simulink model "Virtual_Exhaust_Aftertreatment_System_Model"  (R2016b)
settings: Solver=FixedStepDiscrete  StartTime=0.0  StopTime=inf  FixedStep=VirtExhATSysMdl.tiSimnTiStep_C  RelTol=1e-3  EnableMultiTasking=on
undefined symbols (not defined in the file or in its folder): VirtExhATSysMdl
libraries: simulink x1
settings Model: Creator=m01wolf  LastModifiedBy=m01wolf
settings DataIOCC: SaveFormat=StructureWithTime  SaveOutput=off  DSMLogging=off  VisualizeSimOutput=off  SaveTime=off  SignalLoggingName=Results
settings OptimizationCC: BlockReduction=off  ConditionallyExecuteInputs=off  LifeSpan=inf
settings DebuggingCC: AllowSymbolicDim=off  SFUnexpectedBacktrackingDiag=warning  SFNoUnconditionalDefaultTransitionDiag=warning  SFExecutionAtInitializationDiag=none
settings ModelReferenceCC: ModelReferenceNumInstancesAllowed=Single  PropagateSignalLabelsOutOfModel=off
settings GRTTargetCC: TargetLangStandard=C89/C90 (ANSI)
settings ConfigComp: CovMetricSettings=dw  CovHtmlReporting=on  CovSaveCumulativeToWorkspaceVar=on  CovSaveSingleToWorkspaceVar=on  CovExternalEMLEnable=off

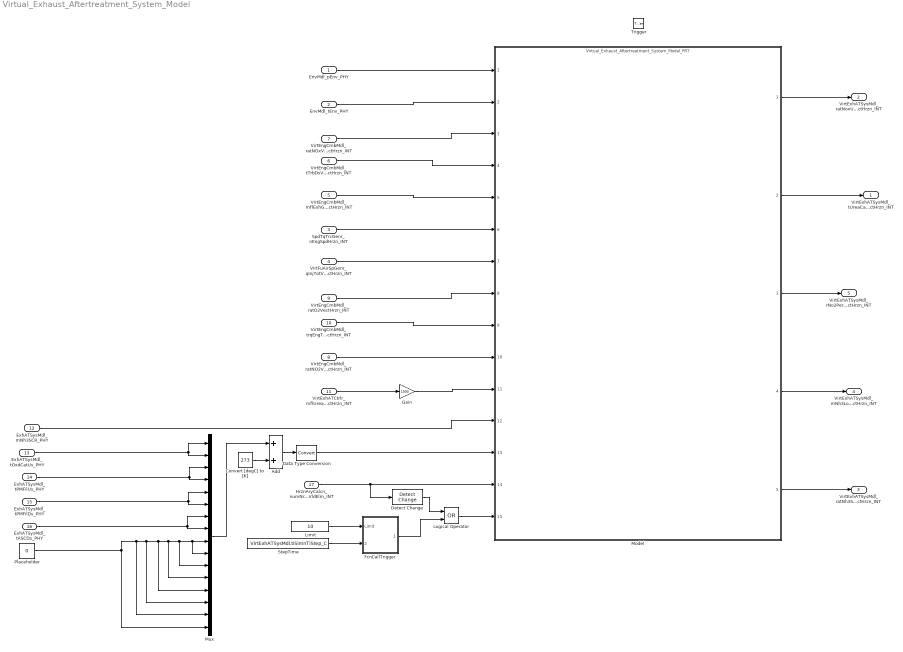
== system Virtual_Exhaust_Aftertreatment_System_Model ==
  EnvMdl_pEnv_PHY : Inport
  EnvMdl_tEnv_PHY : Inport  Port=2
  SpdTqTrcGenr_nEngSpdHrzn_INT : Inport  Port=3  PortDimensions=VirtExhATSysMdl_numHrznSize_CA
  VirtFuAirSpGenr_qInjTotVectHrzn_INT : Inport  Port=4  PortDimensions=VirtExhATSysMdl_numHrznSize_CA
  VirtEngCmbMdl_mflExhGasVectHrzn_INT : Inport  Port=5  PortDimensions=VirtExhATSysMdl_numHrznSize_CA
  VirtEngCmbMdl_tTrbDsVectHrzn_INT : Inport  Port=6  PortDimensions=VirtExhATSysMdl_numHrznSize_CA
  VirtEngCmbMdl_ratNOxVectHrzn_INT : Inport  Port=7  PortDimensions=VirtExhATSysMdl_numHrznSize_CA
  VirtEngCmbMdl_ratNO2VectHrzn_INT : Inport  Port=8  PortDimensions=VirtExhATSysMdl_numHrznSize_CA
  VirtEngCmbMdl_ratO2VectHrzn_INT : Inport  Port=9  PortDimensions=VirtExhATSysMdl_numHrznSize_CA
  VirtEngCmbMdl_trqEngTqOutVectHrzn_INT : Inport  Port=10  PortDimensions=VirtExhATSysMdl_numHrznSize_CA
  VirtExhATCtrlr_mflUreaDesVectHrzn_INT : Inport  Port=11  PortDimensions=VirtExhATSysMdl_numHrznSize_CA
  ExhATSysMdl_mNh3SCR_PHY : Inport  Port=12
  ExhATSysMdl_tOxdCatUs_PHY : Inport  Port=13
  ExhATSysMdl_tPMFilUs_PHY : Inport  Port=14
  ExhATSysMdl_tPMFilDs_PHY : Inport  Port=15
  ExhATSysMdl_tASCDs_PHY : Inport  Port=16
  HrznAryCalcn_numNrHrznVldElm_INT : Inport  Port=17
  Trigger : TriggerPort  TriggerType=function-call  VariantControl=Variant  PortDimensions=1
  Add : Sum
  Convert [degC] to [K] : Constant  Value=273
  Data Type Conversion : DataTypeConversion
  Detect Change : simulink/Logic and Bit Operations/Detect Change  vinit=0  OutDataTypeStr=boolean
  FcnCallTrigger : Subsystem  TreatAsAtomicUnit=on
  Gain : Gain  Gain=1500
  Limit : Constant  Value=10
  Logical Operator : Logic  Operator=OR  AllPortsSameDT=off  OutDataTypeStr=boolean
  Model : ModelReference  ModelNameDialog=Virtual_Exhaust_Aftertreatment_System_Model_PRT.slxp  ModelReferenceVersion=1.99  CopyOfModelProtected=on
  Mux : Mux  Inputs=16
  Placeholder : Constant  Value=0
  StepTime : Constant  Value=VirtExhATSysMdl.tiSimnTiStep_C
  VirtExhATSysMdl_tUreaCatUsVectHrzn_INT : Outport  PortDimensions=VirtExhATSysMdl_numHrznSize_CA
  VirtExhATSysMdl_ratNoxUreaCatDsVectHrzn_INT : Outport  Port=2  PortDimensions=VirtExhATSysMdl_numHrznSize_CA
  VirtExhATSysMdl_ratNh3SnsrDsVectHrzn_INT : Outport  Port=3  PortDimensions=VirtExhATSysMdl_numHrznSize_CA
  VirtExhATSysMdl_mNh3LoadSCRVectHrzn_INT : Outport  Port=4  PortDimensions=VirtExhATSysMdl_numHrznSize_CA
  VirtExhATSysMdl_rNo2PerNoxUreaCatUsVectHrzn_INT : Outport  Port=5  PortDimensions=VirtExhATSysMdl_numHrznSize_CA
  wires:
  EnvMdl_pEnv_PHY/1 -> Model/1
  EnvMdl_tEnv_PHY/1 -> Model/2
  VirtEngCmbMdl_mflExhGasVectHrzn_INT/1 -> Model/5
  ExhATSysMdl_mNh3SCR_PHY/1 -> Model/12
  SpdTqTrcGenr_nEngSpdHrzn_INT/1 -> Model/6
  VirtFuAirSpGenr_qInjTotVectHrzn_INT/1 -> Model/7
  VirtEngCmbMdl_ratNOxVectHrzn_INT/1 -> Model/3
  VirtEngCmbMdl_ratNO2VectHrzn_INT/1 -> Model/10
  VirtEngCmbMdl_ratO2VectHrzn_INT/1 -> Model/8
  VirtEngCmbMdl_tTrbDsVectHrzn_INT/1 -> Model/4
  VirtEngCmbMdl_trqEngTqOutVectHrzn_INT/1 -> Model/9
  VirtExhATCtrlr_mflUreaDesVectHrzn_INT/1 -> Gain/1
  ExhATSysMdl_tOxdCatUs_PHY/1 -> Mux/1, Mux/2
  ExhATSysMdl_tPMFilUs_PHY/1 -> Mux/3, Mux/4
  ExhATSysMdl_tPMFilDs_PHY/1 -> Mux/5, Mux/6
  ExhATSysMdl_tASCDs_PHY/1 -> Mux/7, Mux/8
  Mux/1 -> Add/1
  Convert [degC] to [K]/1 -> Add/2
  Add/1 -> Data Type Conversion/1
  Placeholder/1 -> Mux/15, Mux/14, Mux/13, Mux/12, Mux/11, Mux/10, Mux/9, Mux/16
  Data Type Conversion/1 -> Model/13
  HrznAryCalcn_numNrHrznVldElm_INT/1 -> Detect Change/1, Model/14
  Model/5 -> VirtExhATSysMdl_ratNh3SnsrDsVectHrzn_INT/1
  Model/4 -> VirtExhATSysMdl_mNh3LoadSCRVectHrzn_INT/1
  Model/3 -> VirtExhATSysMdl_rNo2PerNoxUreaCatUsVectHrzn_INT/1
  Model/2 -> VirtExhATSysMdl_tUreaCatUsVectHrzn_INT/1
  Model/1 -> VirtExhATSysMdl_ratNoxUreaCatDsVectHrzn_INT/1
  Limit/1 -> FcnCallTrigger/1(Limit)
  StepTime/1 -> FcnCallTrigger/2(StepTime)
  FcnCallTrigger/1(Trigger) -> Logical Operator/2
  Gain/1 -> Model/11
  Logical Operator/1 -> Model/15
  Detect Change/1 -> Logical Operator/1

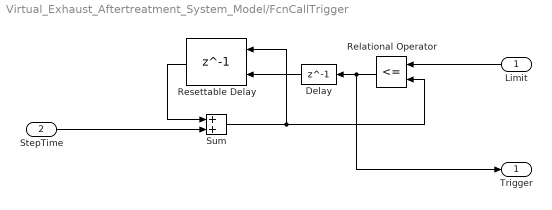
== system Virtual_Exhaust_Aftertreatment_System_Model/FcnCallTrigger ==
  Limit : Inport
  StepTime : Inport  Port=2
  Delay : Delay  DelayLength=1  InitialCondition=1
  Relational Operator : RelationalOperator  Operator=<=  OutDataTypeStr=boolean  RndMeth=Simplest
  Resettable Delay : Delay  DelayLength=1  InitialCondition=0  ExternalReset=Rising
      settings: InputPortMap=u0,r5
  Sum : Sum
  Trigger : Outport
  wires:
  StepTime/1 -> Sum/2
  Delay/1 -> Resettable Delay/2
  Resettable Delay/1 -> Sum/1
  Sum/1 -> Relational Operator/2, Resettable Delay/1
  Limit/1 -> Relational Operator/1
  Relational Operator/1 -> Trigger/1, Delay/1
